simulink model "kalman_estimate_MM"  (R2018b)
settings: Solver=FixedStepAuto  StartTime=0.0  StopTime=500  FixedStep=0.02  RelTol=1e-3
values from neighbouring files (symbols this model uses):
  D = randn(num_output,num_control)    [Com_of_linear_model_calculate.m]    (also in Copy_of_linear_model_calculate.m; D.mat = [0 0 0.00507528406191 0.0236369284061 0.221173094143 0.00198; LINEAR.m = randn(8,1)*10; MM_HKF.m = reshape(out(A_l+B_l+C_l+1:A_l+B_l+C_l+D_l),size_D))
undefined symbols (not defined in the file or in its folder): act_piece, com_piece, piece, sigbuilder_block
libraries: sharedschedule x467, dspsigattribs x44, commchan3 x1
(part 3 of 5)

== system kalman_estimate_MM/HKF8 ==
  In3 : Inport
  In4 : Inport  Port=2
  x_obem : Inport  Port=3
  y_obem : Inport  Port=4
  A : sharedschedule/Interpolate Matrix(x)   matrix=piece.A  aMode=aMode
      settings: SourceProductName=Aerospace Blockset  SourceProductBaseCode=AE
  Add : Sum
  B : sharedschedule/Interpolate Matrix(x)   matrix=piece.B  aMode=aMode
      settings: SourceProductName=Aerospace Blockset  SourceProductBaseCode=AE
  C : sharedschedule/Interpolate Matrix(x)   matrix=piece.C  aMode=aMode
      settings: SourceProductName=Aerospace Blockset  SourceProductBaseCode=AE
  D : sharedschedule/Interpolate Matrix(x)   matrix=piece.D  aMode=aMode
      settings: SourceProductName=Aerospace Blockset  SourceProductBaseCode=AE
  K_s : sharedschedule/Interpolate Matrix(x)   matrix=piece.K_s  aMode=aMode
      settings: SourceProductName=Aerospace Blockset  SourceProductBaseCode=AE
  L : sharedschedule/Interpolate Matrix(x)   matrix=piece.L  aMode=aMode
      settings: SourceProductName=Aerospace Blockset  SourceProductBaseCode=AE
  M : sharedschedule/Interpolate Matrix(x)   matrix=piece.M  aMode=aMode
      settings: SourceProductName=Aerospace Blockset  SourceProductBaseCode=AE
  Prelookup : PreLookup  BreakpointsData=piece.Nl  BreakpointObject=Nl  ExtrapMethod=Linear  UseLastBreakpoint=on  DiagnosticForOutOfRangeInput=Warning
  S : sharedschedule/Interpolate Matrix(x)   matrix=piece.S_s  aMode=aMode
      settings: SourceProductName=Aerospace Blockset  SourceProductBaseCode=AE
  Selector : Selector  InputPortWidth=2  IndexOptions=Index vector (dialog)  Indices=[1]  OutputSizes=1
  kalman filter1 : Subsystem
  steadyOutput : sharedschedule/Interpolate Matrix(x)   matrix=piece.steadyOutput  aMode=aMode
      settings: SourceProductName=Aerospace Blockset  SourceProductBaseCode=AE
  steadyState : sharedschedule/Interpolate Matrix(x)   matrix=piece.steadyState  aMode=aMode
      settings: SourceProductName=Aerospace Blockset  SourceProductBaseCode=AE
  steadyinput : sharedschedule/Interpolate Matrix(x)   matrix=piece.steadyInput  aMode=aMode
      settings: SourceProductName=Aerospace Blockset  SourceProductBaseCode=AE
  Out1 : Outport
  Out2 : Outport  Port=2
  wires:
  Prelookup/1 -> S/1, K_s/1, M/1, L/1, steadyState/1, steadyinput/1, steadyOutput/1, D/1, C/1, B/1, A/1
  In4/1 -> kalman filter1/7(P)
  Prelookup/2 -> A/2, steadyState/2, S/2, K_s/2, M/2, L/2, steadyinput/2, steadyOutput/2, D/2, C/2, B/2
  Selector/1 -> Prelookup/1
  L/1 -> kalman filter1/5(L)
  C/1 -> kalman filter1/2(C)
  kalman filter1/1(X_es) -> Selector/1
  A/1 -> kalman filter1/1(A)
  M/1 -> kalman filter1/6(M)
  In3/1 -> kalman filter1/3(x0)
  x_obem/1 -> kalman filter1/4(Xtrim)
  y_obem/1 -> Add/2
  kalman filter1/2(Y_es) -> Add/1, Out1/1
  Add/1 -> Out2/1

== system kalman_estimate_MM/HKF9 ==
  In2 : Inport
  In3 : Inport  Port=2
  In4 : Inport  Port=3
  x_obem : Inport  Port=4
  y_obem : Inport  Port=5
  A : sharedschedule/Interpolate Matrix(x)   matrix=piece.A  aMode=aMode
      settings: SourceProductName=Aerospace Blockset  SourceProductBaseCode=AE
  B : sharedschedule/Interpolate Matrix(x)   matrix=piece.B  aMode=aMode
      settings: SourceProductName=Aerospace Blockset  SourceProductBaseCode=AE
  C : sharedschedule/Interpolate Matrix(x)   matrix=piece.C  aMode=aMode
      settings: SourceProductName=Aerospace Blockset  SourceProductBaseCode=AE
  D : sharedschedule/Interpolate Matrix(x)   matrix=piece.D  aMode=aMode
      settings: SourceProductName=Aerospace Blockset  SourceProductBaseCode=AE
  K_s : sharedschedule/Interpolate Matrix(x)   matrix=piece.K_s  aMode=aMode
      settings: SourceProductName=Aerospace Blockset  SourceProductBaseCode=AE
  L : sharedschedule/Interpolate Matrix(x)   matrix=piece.L  aMode=aMode
      settings: SourceProductName=Aerospace Blockset  SourceProductBaseCode=AE
  M : sharedschedule/Interpolate Matrix(x)   matrix=piece.M  aMode=aMode
      settings: SourceProductName=Aerospace Blockset  SourceProductBaseCode=AE
  MATLAB Function : MATLAB Function  TreatAsAtomicUnit=on
  Minus5 : Sum  Inputs=+-
  Prelookup : PreLookup  BreakpointsData=piece.Nl  BreakpointObject=Nl  ExtrapMethod=Linear  UseLastBreakpoint=on  DiagnosticForOutOfRangeInput=Warning
  S : sharedschedule/Interpolate Matrix(x)   matrix=piece.S_s  aMode=aMode
      settings: SourceProductName=Aerospace Blockset  SourceProductBaseCode=AE
  Selector : Selector  InputPortWidth=2  IndexOptions=Index vector (dialog)  Indices=[1]  OutputSizes=1
  kalman filter1 : Subsystem
  steadyOutput : sharedschedule/Interpolate Matrix(x)   matrix=piece.steadyOutput  aMode=aMode
      settings: SourceProductName=Aerospace Blockset  SourceProductBaseCode=AE
  steadyState : sharedschedule/Interpolate Matrix(x)   matrix=piece.steadyState  aMode=aMode
      settings: SourceProductName=Aerospace Blockset  SourceProductBaseCode=AE
  steadyinput : sharedschedule/Interpolate Matrix(x)   matrix=piece.steadyInput  aMode=aMode
      settings: SourceProductName=Aerospace Blockset  SourceProductBaseCode=AE
  Out1 : Outport
  Out2 : Outport  Port=2
  Out3 : Outport  Port=3
  wires:
  S/1 -> MATLAB Function/2(S)
  kalman filter1/3(Y_error) -> Out2/1, MATLAB Function/1(err)
  MATLAB Function/1(y) -> Out3/1
  Prelookup/1 -> S/1, K_s/1, M/1, L/1, steadyState/1, steadyinput/1, steadyOutput/1, D/1, C/1, B/1, A/1
  In4/1 -> kalman filter1/9(P)
  Prelookup/2 -> A/2, steadyState/2, S/2, K_s/2, M/2, L/2, steadyinput/2, steadyOutput/2, D/2, C/2, B/2
  Selector/1 -> Prelookup/1
  L/1 -> kalman filter1/7(L)
  C/1 -> kalman filter1/2(C)
  Minus5/1 -> kalman filter1/5(Y)
  kalman filter1/2(Y_es) -> Out1/1
  kalman filter1/1(X_es) -> Selector/1
  K_s/1 -> kalman filter1/3(K)
  A/1 -> kalman filter1/1(A)
  M/1 -> kalman filter1/8(M)
  In3/1 -> kalman filter1/4(x0)
  In2/1 -> Minus5/1
  y_obem/1 -> Minus5/2
  x_obem/1 -> kalman filter1/6(Xtrim)

== system kalman_estimate_MM/PIECE kalman ==
  In1 : Inport
  In2 : Inport  Port=2
  In3 : Inport  Port=3
  In4 : Inport  Port=4
  A : sharedschedule/Interpolate Matrix(x)   matrix=piece.A  aMode=aMode
      settings: SourceProductName=Aerospace Blockset  SourceProductBaseCode=AE
  B : sharedschedule/Interpolate Matrix(x)   matrix=piece.B  aMode=aMode
      settings: SourceProductName=Aerospace Blockset  SourceProductBaseCode=AE
  C : sharedschedule/Interpolate Matrix(x)   matrix=piece.C  aMode=aMode
      settings: SourceProductName=Aerospace Blockset  SourceProductBaseCode=AE
  D : sharedschedule/Interpolate Matrix(x)   matrix=piece.D  aMode=aMode
      settings: SourceProductName=Aerospace Blockset  SourceProductBaseCode=AE
  K_s : sharedschedule/Interpolate Matrix(x)   matrix=piece.K_s  aMode=aMode
      settings: SourceProductName=Aerospace Blockset  SourceProductBaseCode=AE
  L : sharedschedule/Interpolate Matrix(x)   matrix=piece.L  aMode=aMode
      settings: SourceProductName=Aerospace Blockset  SourceProductBaseCode=AE
  M : sharedschedule/Interpolate Matrix(x)   matrix=piece.M  aMode=aMode
      settings: SourceProductName=Aerospace Blockset  SourceProductBaseCode=AE
  Minus1 : Sum  Inputs=+-
  Minus5 : Sum  Inputs=+-
  Prelookup : PreLookup  BreakpointsData=piece.Nl  BreakpointObject=Nl  ExtrapMethod=Linear  UseLastBreakpoint=on  DiagnosticForOutOfRangeInput=Warning
  S : sharedschedule/Interpolate Matrix(x)   matrix=piece.S_s  aMode=aMode
      settings: SourceProductName=Aerospace Blockset  SourceProductBaseCode=AE
  Selector : Selector  InputPortWidth=2  IndexOptions=Index vector (dialog)  Indices=[1]  OutputSizes=1
  kalman filter1 : Subsystem
  steadyOutput : sharedschedule/Interpolate Matrix(x)   matrix=piece.steadyOutput  aMode=aMode
      settings: SourceProductName=Aerospace Blockset  SourceProductBaseCode=AE
  steadyState : sharedschedule/Interpolate Matrix(x)   matrix=piece.steadyState  aMode=aMode
      settings: SourceProductName=Aerospace Blockset  SourceProductBaseCode=AE
  steadyinput : sharedschedule/Interpolate Matrix(x)   matrix=piece.steadyInput  aMode=aMode
      settings: SourceProductName=Aerospace Blockset  SourceProductBaseCode=AE
  Out1 : Outport
  Out2 : Outport  Port=2
  wires:
  kalman filter1/3(Y_error) -> Out2/1
  In1/1 -> Minus1/1
  In2/1 -> Minus5/1
  In3/1 -> kalman filter1/6(x0)
  M/1 -> kalman filter1/11(M)
  A/1 -> kalman filter1/1(A)
  steadyOutput/1 -> Minus5/2
  K_s/1 -> kalman filter1/5(K)
  steadyinput/1 -> Minus1/2
  kalman filter1/1(X_es) -> Selector/1
  Minus1/1 -> kalman filter1/8(U)
  kalman filter1/2(Y_es) -> Out1/1
  Minus5/1 -> kalman filter1/7(Y)
  C/1 -> kalman filter1/3(C)
  L/1 -> kalman filter1/10(L)
  steadyState/1 -> kalman filter1/9(Xtrim)
  Selector/1 -> Prelookup/1
  Prelookup/2 -> B/2, C/2, D/2, steadyOutput/2, steadyinput/2, L/2, M/2, K_s/2, S/2, steadyState/2, A/2
  B/1 -> kalman filter1/2(B)
  In4/1 -> kalman filter1/12(P)
  Prelookup/1 -> A/1, B/1, C/1, D/1, steadyOutput/1, steadyinput/1, steadyState/1, L/1, M/1, K_s/1, S/1
  D/1 -> kalman filter1/4(D)

== system kalman_estimate_MM/PIECE kalman1 ==
  u : Inport
  y : Inport  Port=2
  x0 : Inport  Port=3
  hp : Inport  Port=4
  A : sharedschedule/Interpolate Matrix(x)   matrix=piece.A  aMode=aMode
      settings: SourceProductName=Aerospace Blockset  SourceProductBaseCode=AE
  B : sharedschedule/Interpolate Matrix(x)   matrix=piece.B  aMode=aMode
      settings: SourceProductName=Aerospace Blockset  SourceProductBaseCode=AE
  C : sharedschedule/Interpolate Matrix(x)   matrix=piece.C  aMode=aMode
      settings: SourceProductName=Aerospace Blockset  SourceProductBaseCode=AE
  D : sharedschedule/Interpolate Matrix(x)   matrix=piece.D  aMode=aMode
      settings: SourceProductName=Aerospace Blockset  SourceProductBaseCode=AE
  K_s : sharedschedule/Interpolate Matrix(x)   matrix=piece.K_s  aMode=aMode
      settings: SourceProductName=Aerospace Blockset  SourceProductBaseCode=AE
  L : sharedschedule/Interpolate Matrix(x)   matrix=piece.L  aMode=aMode
      settings: SourceProductName=Aerospace Blockset  SourceProductBaseCode=AE
  M : sharedschedule/Interpolate Matrix(x)   matrix=piece.M  aMode=aMode
      settings: SourceProductName=Aerospace Blockset  SourceProductBaseCode=AE
  MATLAB Function : MATLAB Function  TreatAsAtomicUnit=on
  Minus1 : Sum  Inputs=+-
  Minus5 : Sum  Inputs=+-
  Prelookup : PreLookup  BreakpointsData=piece.Nl  BreakpointObject=Nl  ExtrapMethod=Linear  UseLastBreakpoint=on  DiagnosticForOutOfRangeInput=Warning
  S : sharedschedule/Interpolate Matrix(x)   matrix=piece.S_s  aMode=aMode
      settings: SourceProductName=Aerospace Blockset  SourceProductBaseCode=AE
  Selector : Selector  InputPortWidth=2  IndexOptions=Index vector (dialog)  Indices=[1]  OutputSizes=1
  kalman filter1 : Subsystem
  steadyOutput : sharedschedule/Interpolate Matrix(x)   matrix=piece.steadyOutput  aMode=aMode
      settings: SourceProductName=Aerospace Blockset  SourceProductBaseCode=AE
  steadyState : sharedschedule/Interpolate Matrix(x)   matrix=piece.steadyState  aMode=aMode
      settings: SourceProductName=Aerospace Blockset  SourceProductBaseCode=AE
  steadyinput : sharedschedule/Interpolate Matrix(x)   matrix=piece.steadyInput  aMode=aMode
      settings: SourceProductName=Aerospace Blockset  SourceProductBaseCode=AE
  Out1 : Outport
  Out2 : Outport  Port=2
  Out3 : Outport  Port=3
  wires:
  u/1 -> Minus1/1
  y/1 -> Minus5/1
  x0/1 -> kalman filter1/6(x0)
  M/1 -> kalman filter1/11(M)
  A/1 -> kalman filter1/1(A)
  steadyOutput/1 -> Minus5/2
  K_s/1 -> kalman filter1/5(K)
  steadyinput/1 -> Minus1/2
  kalman filter1/1(X_es) -> Selector/1
  Minus1/1 -> kalman filter1/8(U)
  kalman filter1/2(Y_es) -> Out1/1
  Minus5/1 -> kalman filter1/7(Y)
  C/1 -> kalman filter1/3(C)
  L/1 -> kalman filter1/10(L)
  steadyState/1 -> kalman filter1/9(Xtrim)
  Selector/1 -> Prelookup/1
  Prelookup/2 -> B/2, C/2, D/2, steadyOutput/2, steadyinput/2, L/2, M/2, K_s/2, S/2, steadyState/2, A/2
  B/1 -> kalman filter1/2(B)
  hp/1 -> kalman filter1/12(P)
  Prelookup/1 -> A/1, B/1, C/1, D/1, steadyOutput/1, steadyinput/1, steadyState/1, L/1, M/1, K_s/1, S/1
  D/1 -> kalman filter1/4(D)
  S/1 -> MATLAB Function/2(S)
  kalman filter1/3(Y_error) -> MATLAB Function/1(err), Out2/1
  MATLAB Function/1(y) -> Out3/1

== system kalman_estimate_MM/PWL ==
  In1 : Inport
  In3 : Inport  Port=2
  In4 : Inport  Port=3
  A : sharedschedule/Interpolate Matrix(x)   matrix=piece.A  aMode=aMode
      settings: SourceProductName=Aerospace Blockset  SourceProductBaseCode=AE
  Add : Sum
  B : sharedschedule/Interpolate Matrix(x)   matrix=piece.B  aMode=aMode
      settings: SourceProductName=Aerospace Blockset  SourceProductBaseCode=AE
  C : sharedschedule/Interpolate Matrix(x)   matrix=piece.C  aMode=aMode
      settings: SourceProductName=Aerospace Blockset  SourceProductBaseCode=AE
  D : sharedschedule/Interpolate Matrix(x)   matrix=piece.D  aMode=aMode
      settings: SourceProductName=Aerospace Blockset  SourceProductBaseCode=AE
  K_s : sharedschedule/Interpolate Matrix(x)   matrix=piece.K_s  aMode=aMode
      settings: SourceProductName=Aerospace Blockset  SourceProductBaseCode=AE
  L : sharedschedule/Interpolate Matrix(x)   matrix=piece.L  aMode=aMode
      settings: SourceProductName=Aerospace Blockset  SourceProductBaseCode=AE
  M : sharedschedule/Interpolate Matrix(x)   matrix=piece.M  aMode=aMode
      settings: SourceProductName=Aerospace Blockset  SourceProductBaseCode=AE
  Minus1 : Sum  Inputs=+-
  Prelookup : PreLookup  BreakpointsData=piece.Nl  BreakpointObject=Nl  ExtrapMethod=Linear  UseLastBreakpoint=on  DiagnosticForOutOfRangeInput=Warning
  S : sharedschedule/Interpolate Matrix(x)   matrix=piece.S_s  aMode=aMode
      settings: SourceProductName=Aerospace Blockset  SourceProductBaseCode=AE
  Selector : Selector  InputPortWidth=2  IndexOptions=Index vector (dialog)  Indices=[1]  OutputSizes=1
  kalman filter1 : Subsystem
  steadyOutput : sharedschedule/Interpolate Matrix(x)   matrix=piece.steadyOutput  aMode=aMode
      settings: SourceProductName=Aerospace Blockset  SourceProductBaseCode=AE
  steadyState : sharedschedule/Interpolate Matrix(x)   matrix=piece.steadyState  aMode=aMode
      settings: SourceProductName=Aerospace Blockset  SourceProductBaseCode=AE
  steadyinput : sharedschedule/Interpolate Matrix(x)   matrix=piece.steadyInput  aMode=aMode
      settings: SourceProductName=Aerospace Blockset  SourceProductBaseCode=AE
  Out1 : Outport
  Out2 : Outport  Port=2
  wires:
  D/1 -> kalman filter1/4(D)
  Prelookup/1 -> S/1, K_s/1, M/1, L/1, steadyState/1, steadyinput/1, steadyOutput/1, D/1, C/1, B/1, A/1
  In4/1 -> kalman filter1/11(P)
  B/1 -> kalman filter1/2(B)
  Prelookup/2 -> A/2, steadyState/2, S/2, K_s/2, M/2, L/2, steadyinput/2, steadyOutput/2, D/2, C/2, B/2
  Selector/1 -> Prelookup/1
  steadyState/1 -> kalman filter1/8(Xtrim)
  L/1 -> kalman filter1/9(L)
  C/1 -> kalman filter1/3(C)
  kalman filter1/2(Y_es) -> Add/1, Out1/1
  Minus1/1 -> kalman filter1/7(U)
  kalman filter1/1(X_es) -> Selector/1
  steadyinput/1 -> Minus1/2
  K_s/1 -> kalman filter1/5(K)
  A/1 -> kalman filter1/1(A)
  M/1 -> kalman filter1/10(M)
  In3/1 -> kalman filter1/6(x0)
  In1/1 -> Minus1/1
  steadyOutput/1 -> Add/2
  Add/1 -> Out2/1

== system kalman_estimate_MM/Signal Builder ==
  Demux : Demux  Tag=STV Demux  Outputs=6
  FromWs : FromWorkspace  Tag=STV FromWs  VariableName=tuvar  SampleTime=0
      SigBuilderData=|
      | common.afterFinalStr = 'Extrapolate'
      | common.sampleTime = 0
      | dataSet.timeRange = [0 500]
      | dataSet.name = 'Group 1'
      | sbobj.Groups.Name = 'Group 1'
      | sbobj.Groups.Signals(1).Name = 'Signal 2'
      | sbobj.Groups.Signals(1).XData = [0 120 120 500]
      | sbobj.Groups.Signals(1).YData = [0 0 -0.02 -0.02]
      | sbobj.Groups.Signals(2).Name = 'Signal 3'
      | sbobj.Groups.Signals(2).XData = [0 135 170 500]
      | sbobj.Groups.Signals(2).YData = [0 0 0 0]
      | sbobj.Groups.Signals(3).Name = 'Signal 4'
      | sbobj.Groups.Signals(3).XData = [0 135 170 500]
      | sbobj.Groups.Signals(3).YData = [0 0 0 0]
      | sbobj.Groups.Signals(4).Name = 'Signal 1'
      | sbobj.Groups.Signals(4).XData = [0 135 170 500]
      | sbobj.Groups.Signals(4).YData = [0 0 0 0]
      | sbobj.Groups.Signals(5).Name = 'Signal 5'
      | sbobj.Groups.Signals(5).XData = [0 135 170 500]
      | sbobj.Groups.Signals(5).YData = [0 0 0 0]
      | sbobj.Groups.Signals(6).Name = 'Signal 6'
      | sbobj.Groups.Signals(6).XData = [0 135 170 500]
      | sbobj.Groups.Signals(6).YData = [0 0 0 0]
      | sbobj.Groups.TimeRange = [0 500]
  Signal 2 : Outport  Tag=STV Outport
  Signal 3 : Outport  Tag=STV Outport  Port=2
  Signal 4 : Outport  Tag=STV Outport  Port=3
  Signal 1 : Outport  Tag=STV Outport  Port=4
  Signal 5 : Outport  Tag=STV Outport  Port=5
  Signal 6 : Outport  Tag=STV Outport  Port=6
  wires:
  FromWs/1 -> Demux/1
  Demux/1 -> Signal 2/1
  Demux/2 -> Signal 3/1
  Demux/3 -> Signal 4/1
  Demux/4 -> Signal 1/1
  Demux/5 -> Signal 5/1
  Demux/6 -> Signal 6/1

== system kalman_estimate_MM/Signal Builder1 ==
  Demux : Demux  Tag=STV Demux  Outputs=6
  FromWs : FromWorkspace  Tag=STV FromWs  VariableName=tuvar  SampleTime=0
      SigBuilderData=|
      | common.afterFinalStr = 'Extrapolate'
      | common.sampleTime = 0
      | dataSet.timeRange = [0 500]
      | dataSet.name = 'Group 1'
      | sbobj.Groups.Name = 'Group 1'
      | sbobj.Groups.Signals(1).Name = 'Signal 2'
      | sbobj.Groups.Signals(1).XData = [0 135 170 500]
      | sbobj.Groups.Signals(1).YData = [0 0 0 0]
      | sbobj.Groups.Signals(2).Name = 'Signal 3'
      | sbobj.Groups.Signals(2).XData = [0 50 50 500]
      | sbobj.Groups.Signals(2).YData = [0 0 -0.02 -0.02]
      | sbobj.Groups.Signals(3).Name = 'Signal 4'
      | sbobj.Groups.Signals(3).XData = [0 135 170 500]
      | sbobj.Groups.Signals(3).YData = [0 0 0 0]
      | sbobj.Groups.Signals(4).Name = 'Signal 1'
      | sbobj.Groups.Signals(4).XData = [0 120 120 500]
      | sbobj.Groups.Signals(4).YData = [0 0 -0.02 -0.02]
      | sbobj.Groups.Signals(5).Name = 'Signal 5'
      | sbobj.Groups.Signals(5).XData = [0 200 200 500]
      | sbobj.Groups.Signals(5).YData = [0 0 -0.02 -0.02]
      | sbobj.Groups.Signals(6).Name = 'Signal 6'
      | sbobj.Groups.Signals(6).XData = [0 135 170 500]
      | sbobj.Groups.Signals(6).YData = [0 0 0 0]
      | sbobj.Groups.TimeRange = [0 500]
  Signal 2 : Outport  Tag=STV Outport
  Signal 3 : Outport  Tag=STV Outport  Port=2
  Signal 4 : Outport  Tag=STV Outport  Port=3
  Signal 1 : Outport  Tag=STV Outport  Port=4
  Signal 5 : Outport  Tag=STV Outport  Port=5
  Signal 6 : Outport  Tag=STV Outport  Port=6
  wires:
  Demux/6 -> Signal 6/1
  Demux/5 -> Signal 5/1
  Demux/4 -> Signal 1/1
  Demux/3 -> Signal 4/1
  Demux/2 -> Signal 3/1
  Demux/1 -> Signal 2/1
  FromWs/1 -> Demux/1

== system kalman_estimate_MM/act_PIECE kalman ==
  u : Inport
  y : Inport  Port=2
  x0 : Inport  Port=3
  A : sharedschedule/Interpolate Matrix(x)   matrix=act_piece.A  aMode=aMode
      settings: SourceProductName=Aerospace Blockset  SourceProductBaseCode=AE
  B : sharedschedule/Interpolate Matrix(x)   matrix=act_piece.B  aMode=aMode
      settings: SourceProductName=Aerospace Blockset  SourceProductBaseCode=AE
  C : sharedschedule/Interpolate Matrix(x)   matrix=act_piece.C  aMode=aMode
      settings: SourceProductName=Aerospace Blockset  SourceProductBaseCode=AE
  D : sharedschedule/Interpolate Matrix(x)   matrix=act_piece.D  aMode=aMode
      settings: SourceProductName=Aerospace Blockset  SourceProductBaseCode=AE
  K_s : sharedschedule/Interpolate Matrix(x)   matrix=act_piece.K  aMode=aMode
      settings: SourceProductName=Aerospace Blockset  SourceProductBaseCode=AE
  MATLAB Function : MATLAB Function  TreatAsAtomicUnit=on
  Minus1 : Sum  Inputs=+-
  Minus5 : Sum  Inputs=+-
  Prelookup : PreLookup  BreakpointsData=act_piece.Nl  BreakpointObject=Nl  ExtrapMethod=Linear  UseLastBreakpoint=on  DiagnosticForOutOfRangeInput=Warning
  S : sharedschedule/Interpolate Matrix(x)   matrix=act_piece.S  aMode=aMode
      settings: SourceProductName=Aerospace Blockset  SourceProductBaseCode=AE
  Selector : Selector  InputPortWidth=2  IndexOptions=Index vector (dialog)  Indices=[1]  OutputSizes=1
  kalman filter1 : Subsystem
  steadyOutput : sharedschedule/Interpolate Matrix(x)   matrix=act_piece.steadyOutput  aMode=aMode
      settings: SourceProductName=Aerospace Blockset  SourceProductBaseCode=AE
  steadyState : sharedschedule/Interpolate Matrix(x)   matrix=act_piece.steadyState  aMode=aMode
      settings: SourceProductName=Aerospace Blockset  SourceProductBaseCode=AE
  steadyinput : sharedschedule/Interpolate Matrix(x)   matrix=piece.steadyInput  aMode=aMode
      settings: SourceProductName=Aerospace Blockset  SourceProductBaseCode=AE
  Out1 : Outport
  Out2 : Outport  Port=2
  Out3 : Outport  Port=3
  wires:
  kalman filter1/3(Y_error) -> MATLAB Function/1(err), Out2/1
  u/1 -> Minus1/1
  y/1 -> Minus5/1
  x0/1 -> kalman filter1/6(x0)
  A/1 -> kalman filter1/1(A)
  steadyOutput/1 -> Minus5/2
  K_s/1 -> kalman filter1/5(K)
  steadyinput/1 -> Minus1/2
  kalman filter1/1(X_es) -> Selector/1
  Minus1/1 -> kalman filter1/8(U)
  kalman filter1/2(Y_es) -> Out1/1
  Minus5/1 -> kalman filter1/7(Y)
  C/1 -> kalman filter1/3(C)
  steadyState/1 -> kalman filter1/9(Xtrim)
  Selector/1 -> Prelookup/1
  Prelookup/2 -> B/2, C/2, D/2, steadyOutput/2, steadyinput/2, K_s/2, S/2, steadyState/2, A/2
  B/1 -> kalman filter1/2(B)
  Prelookup/1 -> A/1, B/1, C/1, D/1, steadyOutput/1, steadyinput/1, steadyState/1, S/1, K_s/1
  D/1 -> kalman filter1/4(D)
  S/1 -> MATLAB Function/2(S)
  MATLAB Function/1(y) -> Out3/1

== system kalman_estimate_MM/act_PWL ==
  u : Inport
  x0 : Inport  Port=2
  A : sharedschedule/Interpolate Matrix(x)   matrix=act_piece.A  aMode=aMode
      settings: SourceProductName=Aerospace Blockset  SourceProductBaseCode=AE
  Add : Sum
  B : sharedschedule/Interpolate Matrix(x)   matrix=act_piece.B  aMode=aMode
      settings: SourceProductName=Aerospace Blockset  SourceProductBaseCode=AE
  C : sharedschedule/Interpolate Matrix(x)   matrix=act_piece.C  aMode=aMode
      settings: SourceProductName=Aerospace Blockset  SourceProductBaseCode=AE
  D : sharedschedule/Interpolate Matrix(x)   matrix=act_piece.D  aMode=aMode
      settings: SourceProductName=Aerospace Blockset  SourceProductBaseCode=AE
  K : sharedschedule/Interpolate Matrix(x)   matrix=act_piece.K  aMode=aMode
      settings: SourceProductName=Aerospace Blockset  SourceProductBaseCode=AE
  Minus1 : Sum  Inputs=+-
  Prelookup : PreLookup  BreakpointsData=act_piece.Nl  BreakpointObject=Nl  ExtrapMethod=Linear  UseLastBreakpoint=on  DiagnosticForOutOfRangeInput=Warning
  S : sharedschedule/Interpolate Matrix(x)   matrix=act_piece.S  aMode=aMode
      settings: SourceProductName=Aerospace Blockset  SourceProductBaseCode=AE
  Selector : Selector  InputPortWidth=2  IndexOptions=Index vector (dialog)  Indices=[1]  OutputSizes=1
  kalman filter1 : Subsystem
  steadyOutput : sharedschedule/Interpolate Matrix(x)   matrix=act_piece.steadyOutput  aMode=aMode
      settings: SourceProductName=Aerospace Blockset  SourceProductBaseCode=AE
  steadyState : sharedschedule/Interpolate Matrix(x)   matrix=act_piece.steadyState  aMode=aMode
      settings: SourceProductName=Aerospace Blockset  SourceProductBaseCode=AE
  steadyinput : sharedschedule/Interpolate Matrix(x)   matrix=act_piece.steadyInput  aMode=aMode
      settings: SourceProductName=Aerospace Blockset  SourceProductBaseCode=AE
  Out1 : Outport
  Out2 : Outport  Port=2
  wires:
  Add/1 -> Out2/1
  steadyOutput/1 -> Add/2
  u/1 -> Minus1/1
  x0/1 -> kalman filter1/5(x0)
  A/1 -> kalman filter1/1(A)
  steadyinput/1 -> Minus1/2
  kalman filter1/1(X_es) -> Selector/1
  Minus1/1 -> kalman filter1/6(U)
  kalman filter1/2(Y_es) -> Out1/1, Add/1
  C/1 -> kalman filter1/3(C)
  steadyState/1 -> kalman filter1/7(Xtrim)
  Selector/1 -> Prelookup/1
  Prelookup/2 -> B/2, C/2, D/2, steadyOutput/2, steadyinput/2, K/2, S/2, steadyState/2, A/2
  B/1 -> kalman filter1/2(B)
  Prelookup/1 -> A/1, B/1, C/1, D/1, steadyOutput/1, steadyinput/1, steadyState/1, K/1, S/1
  D/1 -> kalman filter1/4(D)

== system kalman_estimate_MM/act_PWL_model ==
  u : Inport
  x0 : Inport  Port=2
  A : sharedschedule/Interpolate Matrix(x)   matrix=act_piece.A  aMode=aMode
      settings: SourceProductName=Aerospace Blockset  SourceProductBaseCode=AE
  Add : Sum
  B : sharedschedule/Interpolate Matrix(x)   matrix=act_piece.B  aMode=aMode
      settings: SourceProductName=Aerospace Blockset  SourceProductBaseCode=AE
  C : sharedschedule/Interpolate Matrix(x)   matrix=act_piece.C  aMode=aMode
      settings: SourceProductName=Aerospace Blockset  SourceProductBaseCode=AE
  D : sharedschedule/Interpolate Matrix(x)   matrix=act_piece.D  aMode=aMode
      settings: SourceProductName=Aerospace Blockset  SourceProductBaseCode=AE
  K : sharedschedule/Interpolate Matrix(x)   matrix=act_piece.K  aMode=aMode
      settings: SourceProductName=Aerospace Blockset  SourceProductBaseCode=AE
  Minus1 : Sum  Inputs=+-
  Prelookup : PreLookup  BreakpointsData=piece.Nl  BreakpointObject=Nl  ExtrapMethod=Linear  UseLastBreakpoint=on  DiagnosticForOutOfRangeInput=Warning
  S : sharedschedule/Interpolate Matrix(x)   matrix=act_piece.S  aMode=aMode
      settings: SourceProductName=Aerospace Blockset  SourceProductBaseCode=AE
  Selector : Selector  InputPortWidth=2  IndexOptions=Index vector (dialog)  Indices=[1]  OutputSizes=1
  kalman filter1 : Subsystem
  steadyOutput : sharedschedule/Interpolate Matrix(x)   matrix=act_piece.steadyOutput  aMode=aMode
      settings: SourceProductName=Aerospace Blockset  SourceProductBaseCode=AE
  steadyState : sharedschedule/Interpolate Matrix(x)   matrix=act_piece.steadyState  aMode=aMode
      settings: SourceProductName=Aerospace Blockset  SourceProductBaseCode=AE
  steadyinput : sharedschedule/Interpolate Matrix(x)   matrix=piece.steadyInput  aMode=aMode
      settings: SourceProductName=Aerospace Blockset  SourceProductBaseCode=AE
  Out1 : Outport
  Out2 : Outport  Port=2
  wires:
  D/1 -> kalman filter1/4(D)
  Prelookup/1 -> S/1, K/1, steadyState/1, steadyinput/1, steadyOutput/1, D/1, C/1, B/1, A/1
  B/1 -> kalman filter1/2(B)
  Prelookup/2 -> A/2, steadyState/2, S/2, K/2, steadyinput/2, steadyOutput/2, D/2, C/2, B/2
  Selector/1 -> Prelookup/1
  steadyState/1 -> kalman filter1/7(Xtrim)
  C/1 -> kalman filter1/3(C)
  kalman filter1/2(Y_es) -> Add/1, Out1/1
  Minus1/1 -> kalman filter1/6(U)
  kalman filter1/1(X_es) -> Selector/1
  steadyinput/1 -> Minus1/2
  A/1 -> kalman filter1/1(A)
  x0/1 -> kalman filter1/5(x0)
  u/1 -> Minus1/1
  steadyOutput/1 -> Add/2
  Add/1 -> Out2/1

== system kalman_estimate_MM/com_PIECE kalman ==
  u : Inport
  y : Inport  Port=2
  x0 : Inport  Port=3
  A : sharedschedule/Interpolate Matrix(x)   matrix=com_piece.A  aMode=aMode
      settings: SourceProductName=Aerospace Blockset  SourceProductBaseCode=AE
  B : sharedschedule/Interpolate Matrix(x)   matrix=com_piece.B  aMode=aMode
      settings: SourceProductName=Aerospace Blockset  SourceProductBaseCode=AE
  C : sharedschedule/Interpolate Matrix(x)   matrix=com_piece.C  aMode=aMode
      settings: SourceProductName=Aerospace Blockset  SourceProductBaseCode=AE
  D : sharedschedule/Interpolate Matrix(x)   matrix=com_piece.D  aMode=aMode
      settings: SourceProductName=Aerospace Blockset  SourceProductBaseCode=AE
  K_s : sharedschedule/Interpolate Matrix(x)   matrix=com_piece.K  aMode=aMode
      settings: SourceProductName=Aerospace Blockset  SourceProductBaseCode=AE
  MATLAB Function : MATLAB Function  TreatAsAtomicUnit=on
  Minus1 : Sum  Inputs=+-
  Minus5 : Sum  Inputs=+-
  Prelookup : PreLookup  BreakpointsData=com_piece.Nl  BreakpointObject=Nl  ExtrapMethod=Linear  UseLastBreakpoint=on  DiagnosticForOutOfRangeInput=Warning
  S : sharedschedule/Interpolate Matrix(x)   matrix=com_piece.S  aMode=aMode
      settings: SourceProductName=Aerospace Blockset  SourceProductBaseCode=AE
  Selector : Selector  InputPortWidth=2  IndexOptions=Index vector (dialog)  Indices=[1]  OutputSizes=1
  kalman filter1 : Subsystem
  steadyOutput : sharedschedule/Interpolate Matrix(x)   matrix=com_piece.steadyOutput  aMode=aMode
      settings: SourceProductName=Aerospace Blockset  SourceProductBaseCode=AE
  steadyState : sharedschedule/Interpolate Matrix(x)   matrix=com_piece.steadyState  aMode=aMode
      settings: SourceProductName=Aerospace Blockset  SourceProductBaseCode=AE
  steadyinput : sharedschedule/Interpolate Matrix(x)   matrix=com_piece.steadyInput  aMode=aMode
      settings: SourceProductName=Aerospace Blockset  SourceProductBaseCode=AE
  Out1 : Outport
  Out2 : Outport  Port=2
  Out3 : Outport  Port=3
  wires:
  kalman filter1/3(Y_error) -> MATLAB Function/1(err), Out2/1
  u/1 -> Minus1/1
  y/1 -> Minus5/1
  x0/1 -> kalman filter1/6(x0)
  A/1 -> kalman filter1/1(A)
  steadyOutput/1 -> Minus5/2
  K_s/1 -> kalman filter1/5(K)
  steadyinput/1 -> Minus1/2
  kalman filter1/1(X_es) -> Selector/1
  Minus1/1 -> kalman filter1/8(U)
  kalman filter1/2(Y_es) -> Out1/1
  Minus5/1 -> kalman filter1/7(Y)
  C/1 -> kalman filter1/3(C)
  steadyState/1 -> kalman filter1/9(Xtrim)
  Selector/1 -> Prelookup/1
  Prelookup/2 -> B/2, C/2, D/2, steadyOutput/2, steadyinput/2, K_s/2, S/2, steadyState/2, A/2
  B/1 -> kalman filter1/2(B)
  Prelookup/1 -> A/1, B/1, C/1, D/1, steadyOutput/1, steadyinput/1, steadyState/1, K_s/1, S/1
  D/1 -> kalman filter1/4(D)
  S/1 -> MATLAB Function/2(S)
  MATLAB Function/1(y) -> Out3/1

== system kalman_estimate_MM/component_PWL ==
  u : Inport
  x0 : Inport  Port=2
  A : sharedschedule/Interpolate Matrix(x)   matrix=com_piece.A  aMode=aMode
      settings: SourceProductName=Aerospace Blockset  SourceProductBaseCode=AE
  Add : Sum
  B : sharedschedule/Interpolate Matrix(x)   matrix=com_piece.B  aMode=aMode
      settings: SourceProductName=Aerospace Blockset  SourceProductBaseCode=AE
  C : sharedschedule/Interpolate Matrix(x)   matrix=com_piece.C  aMode=aMode
      settings: SourceProductName=Aerospace Blockset  SourceProductBaseCode=AE
  D : sharedschedule/Interpolate Matrix(x)   matrix=com_piece.D  aMode=aMode
      settings: SourceProductName=Aerospace Blockset  SourceProductBaseCode=AE
  K : sharedschedule/Interpolate Matrix(x)   matrix=com_piece.K  aMode=aMode
      settings: SourceProductName=Aerospace Blockset  SourceProductBaseCode=AE
  Minus1 : Sum  Inputs=+-
  Prelookup : PreLookup  BreakpointsData=com_piece.Nl  BreakpointObject=Nl  ExtrapMethod=Linear  UseLastBreakpoint=on  DiagnosticForOutOfRangeInput=Warning
  S : sharedschedule/Interpolate Matrix(x)   matrix=com_piece.S  aMode=aMode
      settings: SourceProductName=Aerospace Blockset  SourceProductBaseCode=AE
  Selector : Selector  InputPortWidth=2  IndexOptions=Index vector (dialog)  Indices=[1]  OutputSizes=1
  kalman filter1 : Subsystem
  steadyOutput : sharedschedule/Interpolate Matrix(x)   matrix=com_piece.steadyOutput  aMode=aMode
      settings: SourceProductName=Aerospace Blockset  SourceProductBaseCode=AE
  steadyState : sharedschedule/Interpolate Matrix(x)   matrix=com_piece.steadyState  aMode=aMode
      settings: SourceProductName=Aerospace Blockset  SourceProductBaseCode=AE
  steadyinput : sharedschedule/Interpolate Matrix(x)   matrix=com_piece.steadyInput  aMode=aMode
      settings: SourceProductName=Aerospace Blockset  SourceProductBaseCode=AE
  Out1 : Outport
  Out2 : Outport  Port=2
  wires:
  Add/1 -> Out2/1
  steadyOutput/1 -> Add/2
  u/1 -> Minus1/1
  x0/1 -> kalman filter1/5(x0)
  A/1 -> kalman filter1/1(A)
  steadyinput/1 -> Minus1/2
  kalman filter1/1(X_es) -> Selector/1
  Minus1/1 -> kalman filter1/6(U)
  kalman filter1/2(Y_es) -> Out1/1, Add/1
  C/1 -> kalman filter1/3(C)
  steadyState/1 -> kalman filter1/7(Xtrim)
  Selector/1 -> Prelookup/1
  Prelookup/2 -> B/2, C/2, D/2, steadyOutput/2, steadyinput/2, K/2, S/2, steadyState/2, A/2
  B/1 -> kalman filter1/2(B)
  Prelookup/1 -> A/1, B/1, C/1, D/1, steadyOutput/1, steadyinput/1, steadyState/1, K/1, S/1
  D/1 -> kalman filter1/4(D)

== system kalman_estimate_MM/component_PWL1 ==
  u : Inport
  x0 : Inport  Port=2
  A : sharedschedule/Interpolate Matrix(x)   matrix=com_piece.A  aMode=aMode
      settings: SourceProductName=Aerospace Blockset  SourceProductBaseCode=AE
  Add : Sum
  B : sharedschedule/Interpolate Matrix(x)   matrix=com_piece.B  aMode=aMode
      settings: SourceProductName=Aerospace Blockset  SourceProductBaseCode=AE
  C : sharedschedule/Interpolate Matrix(x)   matrix=com_piece.C  aMode=aMode
      settings: SourceProductName=Aerospace Blockset  SourceProductBaseCode=AE
  D : sharedschedule/Interpolate Matrix(x)   matrix=com_piece.D  aMode=aMode
      settings: SourceProductName=Aerospace Blockset  SourceProductBaseCode=AE
  K : sharedschedule/Interpolate Matrix(x)   matrix=com_piece.K  aMode=aMode
      settings: SourceProductName=Aerospace Blockset  SourceProductBaseCode=AE
  Minus1 : Sum  Inputs=+-
  Prelookup : PreLookup  BreakpointsData=com_piece.Nl  BreakpointObject=Nl  ExtrapMethod=Linear  UseLastBreakpoint=on  DiagnosticForOutOfRangeInput=Warning
  S : sharedschedule/Interpolate Matrix(x)   matrix=com_piece.S  aMode=aMode
      settings: SourceProductName=Aerospace Blockset  SourceProductBaseCode=AE
  Selector : Selector  InputPortWidth=2  IndexOptions=Index vector (dialog)  Indices=[1]  OutputSizes=1
  kalman filter1 : Subsystem
  steadyOutput : sharedschedule/Interpolate Matrix(x)   matrix=com_piece.steadyOutput  aMode=aMode
      settings: SourceProductName=Aerospace Blockset  SourceProductBaseCode=AE
  steadyState : sharedschedule/Interpolate Matrix(x)   matrix=com_piece.steadyState  aMode=aMode
      settings: SourceProductName=Aerospace Blockset  SourceProductBaseCode=AE
  steadyinput : sharedschedule/Interpolate Matrix(x)   matrix=piece.steadyInput  aMode=aMode
      settings: SourceProductName=Aerospace Blockset  SourceProductBaseCode=AE
  Out1 : Outport
  Out2 : Outport  Port=2
  wires:
  Add/1 -> Out2/1
  steadyOutput/1 -> Add/2
  u/1 -> Minus1/1
  x0/1 -> kalman filter1/5(x0)
  A/1 -> kalman filter1/1(A)
  steadyinput/1 -> Minus1/2
  kalman filter1/1(X_es) -> Selector/1
  Minus1/1 -> kalman filter1/6(U)
  kalman filter1/2(Y_es) -> Out1/1, Add/1
  C/1 -> kalman filter1/3(C)
  steadyState/1 -> kalman filter1/7(Xtrim)
  Selector/1 -> Prelookup/1
  Prelookup/2 -> B/2, C/2, D/2, steadyOutput/2, steadyinput/2, K/2, S/2, steadyState/2, A/2
  B/1 -> kalman filter1/2(B)
  Prelookup/1 -> A/1, B/1, C/1, D/1, steadyOutput/1, steadyinput/1, steadyState/1, K/1, S/1
  D/1 -> kalman filter1/4(D)

== system kalman_estimate_MM/health_PWL ==
  In1 : Inport
  In3 : Inport  Port=2
  In4 : Inport  Port=3
  A : sharedschedule/Interpolate Matrix(x)   matrix=piece.A  aMode=aMode
      settings: SourceProductName=Aerospace Blockset  SourceProductBaseCode=AE
  Add : Sum
  B : sharedschedule/Interpolate Matrix(x)   matrix=piece.B  aMode=aMode
      settings: SourceProductName=Aerospace Blockset  SourceProductBaseCode=AE
  C : sharedschedule/Interpolate Matrix(x)   matrix=piece.C  aMode=aMode
      settings: SourceProductName=Aerospace Blockset  SourceProductBaseCode=AE
  D : sharedschedule/Interpolate Matrix(x)   matrix=piece.D  aMode=aMode
      settings: SourceProductName=Aerospace Blockset  SourceProductBaseCode=AE
  K_s : sharedschedule/Interpolate Matrix(x)   matrix=piece.K_s  aMode=aMode
      settings: SourceProductName=Aerospace Blockset  SourceProductBaseCode=AE
  L : sharedschedule/Interpolate Matrix(x)   matrix=piece.L  aMode=aMode
      settings: SourceProductName=Aerospace Blockset  SourceProductBaseCode=AE
  M : sharedschedule/Interpolate Matrix(x)   matrix=piece.M  aMode=aMode
      settings: SourceProductName=Aerospace Blockset  SourceProductBaseCode=AE
  MATLAB Function : MATLAB Function  TreatAsAtomicUnit=on
  Minus1 : Sum  Inputs=+-
  Prelookup : PreLookup  BreakpointsData=piece.Nl  BreakpointObject=Nl  ExtrapMethod=Linear  UseLastBreakpoint=on  DiagnosticForOutOfRangeInput=Warning
  S : sharedschedule/Interpolate Matrix(x)   matrix=piece.S_s  aMode=aMode
      settings: SourceProductName=Aerospace Blockset  SourceProductBaseCode=AE
  Selector : Selector  InputPortWidth=2  IndexOptions=Index vector (dialog)  Indices=[1]  OutputSizes=1
  kalman filter1 : Subsystem
  steadyOutput : sharedschedule/Interpolate Matrix(x)   matrix=piece.steadyOutput  aMode=aMode
      settings: SourceProductName=Aerospace Blockset  SourceProductBaseCode=AE
  steadyState : sharedschedule/Interpolate Matrix(x)   matrix=piece.steadyState  aMode=aMode
      settings: SourceProductName=Aerospace Blockset  SourceProductBaseCode=AE
  steadyinput : sharedschedule/Interpolate Matrix(x)   matrix=piece.steadyInput  aMode=aMode
      settings: SourceProductName=Aerospace Blockset  SourceProductBaseCode=AE
  Out1 : Outport
  Out2 : Outport  Port=2
  wires:
  D/1 -> kalman filter1/4(D)
  Prelookup/1 -> S/1, K_s/1, M/1, L/1, steadyState/1, steadyinput/1, steadyOutput/1, D/1, C/1, B/1, A/1
  In4/1 -> kalman filter1/11(P)
  B/1 -> kalman filter1/2(B)
  Prelookup/2 -> A/2, steadyState/2, S/2, K_s/2, M/2, L/2, steadyinput/2, steadyOutput/2, D/2, C/2, B/2
  Selector/1 -> Prelookup/1
  steadyState/1 -> kalman filter1/8(Xtrim)
  L/1 -> kalman filter1/9(L)
  C/1 -> kalman filter1/3(C)
  kalman filter1/2(Y_es) -> Add/1, Out1/1
  Minus1/1 -> kalman filter1/7(U)
  kalman filter1/1(X_es) -> Selector/1
  steadyinput/1 -> Minus1/2
  K_s/1 -> kalman filter1/5(K)
  A/1 -> kalman filter1/1(A)
  M/1 -> kalman filter1/10(M)
  In3/1 -> kalman filter1/6(x0)
  In1/1 -> Minus1/1
  steadyOutput/1 -> Add/2
  Add/1 -> Out2/1
  S/1 -> MATLAB Function/2(S)

== system kalman_estimate_MM/sen2_PIECE kalman2 ==
  u : Inport
  y : Inport  Port=2
  x0 : Inport  Port=3
  A : sharedschedule/Interpolate Matrix(x)   matrix=sen2_piece.A  aMode=aMode
      settings: SourceProductName=Aerospace Blockset  SourceProductBaseCode=AE
  B : sharedschedule/Interpolate Matrix(x)   matrix=sen2_piece.B  aMode=aMode
      settings: SourceProductName=Aerospace Blockset  SourceProductBaseCode=AE
  C : sharedschedule/Interpolate Matrix(x)   matrix=sen2_piece.C  aMode=aMode
      settings: SourceProductName=Aerospace Blockset  SourceProductBaseCode=AE
  D : sharedschedule/Interpolate Matrix(x)   matrix=sen2_piece.D  aMode=aMode
      settings: SourceProductName=Aerospace Blockset  SourceProductBaseCode=AE
  K_s : sharedschedule/Interpolate Matrix(x)   matrix=sen2_piece.K  aMode=aMode
      settings: SourceProductName=Aerospace Blockset  SourceProductBaseCode=AE
  MATLAB Function : MATLAB Function  TreatAsAtomicUnit=on
  Minus1 : Sum  Inputs=+-
  Minus5 : Sum  Inputs=+-
  Prelookup : PreLookup  BreakpointsData=sen2_piece.Nl  BreakpointObject=Nl  ExtrapMethod=Linear  UseLastBreakpoint=on  DiagnosticForOutOfRangeInput=Warning
  S : sharedschedule/Interpolate Matrix(x)   matrix=sen2_piece.S  aMode=aMode
      settings: SourceProductName=Aerospace Blockset  SourceProductBaseCode=AE
  Selector : Selector  InputPortWidth=2  IndexOptions=Index vector (dialog)  Indices=[1]  OutputSizes=1
  kalman filter1 : Subsystem
  steadyOutput : sharedschedule/Interpolate Matrix(x)   matrix=sen2_piece.steadyOutput  aMode=aMode
      settings: SourceProductName=Aerospace Blockset  SourceProductBaseCode=AE
  steadyState : sharedschedule/Interpolate Matrix(x)   matrix=sen2_piece.steadyState  aMode=aMode
      settings: SourceProductName=Aerospace Blockset  SourceProductBaseCode=AE
  steadyinput : sharedschedule/Interpolate Matrix(x)   matrix=sen2_piece.steadyInput  aMode=aMode
      settings: SourceProductName=Aerospace Blockset  SourceProductBaseCode=AE
  Out1 : Outport
  Out2 : Outport  Port=2
  Out3 : Outport  Port=3
  wires:
  kalman filter1/3(Y_error) -> MATLAB Function/1(err), Out2/1
  u/1 -> Minus1/1
  y/1 -> Minus5/1
  x0/1 -> kalman filter1/6(x0)
  A/1 -> kalman filter1/1(A)
  steadyOutput/1 -> Minus5/2
  K_s/1 -> kalman filter1/5(K)
  steadyinput/1 -> Minus1/2
  kalman filter1/1(X_es) -> Selector/1
  Minus1/1 -> kalman filter1/8(U)
  kalman filter1/2(Y_es) -> Out1/1
  Minus5/1 -> kalman filter1/7(Y)
  C/1 -> kalman filter1/3(C)
  steadyState/1 -> kalman filter1/9(Xtrim)
  Selector/1 -> Prelookup/1
  Prelookup/2 -> B/2, C/2, D/2, steadyOutput/2, steadyinput/2, K_s/2, S/2, steadyState/2, A/2
  B/1 -> kalman filter1/2(B)
  Prelookup/1 -> A/1, B/1, C/1, D/1, steadyOutput/1, steadyinput/1, steadyState/1, K_s/1, S/1
  D/1 -> kalman filter1/4(D)
  S/1 -> MATLAB Function/2(S)
  MATLAB Function/1(y) -> Out3/1

== system kalman_estimate_MM/sen2_PWL ==
  u : Inport
  x0 : Inport  Port=2
  A : sharedschedule/Interpolate Matrix(x)   matrix=sen2_piece.A  aMode=aMode
      settings: SourceProductName=Aerospace Blockset  SourceProductBaseCode=AE
  Add : Sum
  B : sharedschedule/Interpolate Matrix(x)   matrix=sen2_piece.B  aMode=aMode
      settings: SourceProductName=Aerospace Blockset  SourceProductBaseCode=AE
  C : sharedschedule/Interpolate Matrix(x)   matrix=sen2_piece.C  aMode=aMode
      settings: SourceProductName=Aerospace Blockset  SourceProductBaseCode=AE
  D : sharedschedule/Interpolate Matrix(x)   matrix=sen2_piece.D  aMode=aMode
      settings: SourceProductName=Aerospace Blockset  SourceProductBaseCode=AE
  K : sharedschedule/Interpolate Matrix(x)   matrix=sen2_piece.K  aMode=aMode
      settings: SourceProductName=Aerospace Blockset  SourceProductBaseCode=AE
  Minus1 : Sum  Inputs=+-
  Prelookup : PreLookup  BreakpointsData=sen2_piece.Nl  BreakpointObject=Nl  ExtrapMethod=Linear  UseLastBreakpoint=on  DiagnosticForOutOfRangeInput=Warning
  S : sharedschedule/Interpolate Matrix(x)   matrix=sen2_piece.S  aMode=aMode
      settings: SourceProductName=Aerospace Blockset  SourceProductBaseCode=AE
  Selector : Selector  InputPortWidth=2  IndexOptions=Index vector (dialog)  Indices=[1]  OutputSizes=1
  kalman filter1 : Subsystem
  steadyOutput : sharedschedule/Interpolate Matrix(x)   matrix=sen2_piece.steadyOutput  aMode=aMode
      settings: SourceProductName=Aerospace Blockset  SourceProductBaseCode=AE
  steadyState : sharedschedule/Interpolate Matrix(x)   matrix=sen2_piece.steadyState  aMode=aMode
      settings: SourceProductName=Aerospace Blockset  SourceProductBaseCode=AE
  steadyinput : sharedschedule/Interpolate Matrix(x)   matrix=sen2_piece.steadyInput  aMode=aMode
      settings: SourceProductName=Aerospace Blockset  SourceProductBaseCode=AE
  Out1 : Outport
  Out2 : Outport  Port=2
  wires:
  Add/1 -> Out2/1
  steadyOutput/1 -> Add/2
  u/1 -> Minus1/1
  x0/1 -> kalman filter1/5(x0)
  A/1 -> kalman filter1/1(A)
  steadyinput/1 -> Minus1/2
  kalman filter1/1(X_es) -> Selector/1
  Minus1/1 -> kalman filter1/6(U)
  kalman filter1/2(Y_es) -> Out1/1, Add/1
  C/1 -> kalman filter1/3(C)
  steadyState/1 -> kalman filter1/7(Xtrim)
  Selector/1 -> Prelookup/1
  Prelookup/2 -> B/2, D/2, steadyOutput/2, steadyinput/2, K/2, S/2, steadyState/2, C/2, A/2
  B/1 -> kalman filter1/2(B)
  Prelookup/1 -> A/1, B/1, D/1, steadyOutput/1, steadyinput/1, steadyState/1, K/1, S/1, C/1
  D/1 -> kalman filter1/4(D)

== system kalman_estimate_MM/sen3_PIECE kalman1 ==
  u : Inport
  y : Inport  Port=2
  x0 : Inport  Port=3
  A : sharedschedule/Interpolate Matrix(x)   matrix=sen3_piece.A  aMode=aMode
      settings: SourceProductName=Aerospace Blockset  SourceProductBaseCode=AE
  B : sharedschedule/Interpolate Matrix(x)   matrix=sen3_piece.B  aMode=aMode
      settings: SourceProductName=Aerospace Blockset  SourceProductBaseCode=AE
  C : sharedschedule/Interpolate Matrix(x)   matrix=sen3_piece.C  aMode=aMode
      settings: SourceProductName=Aerospace Blockset  SourceProductBaseCode=AE
  Constant : Constant  Value=[0,0,0.03,0,0,0,0,0,0,0]'  VectorParams1D=off
  D : sharedschedule/Interpolate Matrix(x)   matrix=sen3_piece.D  aMode=aMode
      settings: SourceProductName=Aerospace Blockset  SourceProductBaseCode=AE
  K_s : sharedschedule/Interpolate Matrix(x)   matrix=sen3_piece.K  aMode=aMode
      settings: SourceProductName=Aerospace Blockset  SourceProductBaseCode=AE
  MATLAB Function : MATLAB Function  TreatAsAtomicUnit=on
  Minus1 : Sum  Inputs=+-
  Minus2 : Sum
  Minus5 : Sum  Inputs=+-
  Prelookup : PreLookup  BreakpointsData=sen3_piece.Nl  BreakpointObject=Nl  ExtrapMethod=Linear  UseLastBreakpoint=on  DiagnosticForOutOfRangeInput=Warning
  S : sharedschedule/Interpolate Matrix(x)   matrix=sen3_piece.S  aMode=aMode
      settings: SourceProductName=Aerospace Blockset  SourceProductBaseCode=AE
  Selector : Selector  InputPortWidth=2  IndexOptions=Index vector (dialog)  Indices=[1]  OutputSizes=1
  kalman filter1 : Subsystem
  steadyOutput : sharedschedule/Interpolate Matrix(x)   matrix=sen3_piece.steadyOutput  aMode=aMode
      settings: SourceProductName=Aerospace Blockset  SourceProductBaseCode=AE
  steadyState : sharedschedule/Interpolate Matrix(x)   matrix=sen3_piece.steadyState  aMode=aMode
      settings: SourceProductName=Aerospace Blockset  SourceProductBaseCode=AE
  steadyinput : sharedschedule/Interpolate Matrix(x)   matrix=sen3_piece.steadyInput  aMode=aMode
      settings: SourceProductName=Aerospace Blockset  SourceProductBaseCode=AE
  Out1 : Outport
  Out2 : Outport  Port=2
  Out3 : Outport  Port=3
  wires:
  MATLAB Function/1(y) -> Out3/1
  S/1 -> MATLAB Function/2(S)
  D/1 -> kalman filter1/4(D)
  Prelookup/1 -> S/1, K_s/1, steadyState/1, steadyinput/1, steadyOutput/1, D/1, C/1, B/1, A/1
  B/1 -> kalman filter1/2(B)
  Prelookup/2 -> A/2, steadyState/2, S/2, K_s/2, steadyinput/2, steadyOutput/2, D/2, C/2, B/2
  Selector/1 -> Prelookup/1
  steadyState/1 -> kalman filter1/9(Xtrim)
  C/1 -> kalman filter1/3(C)
  Minus5/1 -> kalman filter1/7(Y)
  kalman filter1/2(Y_es) -> Out1/1
  Minus1/1 -> kalman filter1/8(U)
  kalman filter1/1(X_es) -> Selector/1
  steadyinput/1 -> Minus1/2
  K_s/1 -> kalman filter1/5(K)
  A/1 -> kalman filter1/1(A)
  x0/1 -> kalman filter1/6(x0)
  y/1 -> Minus5/1
  u/1 -> Minus1/1
  kalman filter1/3(Y_error) -> Out2/1, MATLAB Function/1(err)
  steadyOutput/1 -> Minus2/1
  Minus2/1 -> Minus5/2
  Constant/1 -> Minus2/2

== system kalman_estimate_MM/sen3_PIECE kalman3 ==
  u : Inport
  y : Inport  Port=2
  x0 : Inport  Port=3
  A : sharedschedule/Interpolate Matrix(x)   matrix=sen3_piece.A  aMode=aMode
      settings: SourceProductName=Aerospace Blockset  SourceProductBaseCode=AE
  B : sharedschedule/Interpolate Matrix(x)   matrix=sen3_piece.B  aMode=aMode
      settings: SourceProductName=Aerospace Blockset  SourceProductBaseCode=AE
  C : sharedschedule/Interpolate Matrix(x)   matrix=sen3_piece.C  aMode=aMode
      settings: SourceProductName=Aerospace Blockset  SourceProductBaseCode=AE
  D : sharedschedule/Interpolate Matrix(x)   matrix=sen3_piece.D  aMode=aMode
      settings: SourceProductName=Aerospace Blockset  SourceProductBaseCode=AE
  K_s : sharedschedule/Interpolate Matrix(x)   matrix=sen3_piece.K  aMode=aMode
      settings: SourceProductName=Aerospace Blockset  SourceProductBaseCode=AE
  MATLAB Function : MATLAB Function  TreatAsAtomicUnit=on
  Minus1 : Sum  Inputs=+-
  Minus5 : Sum  Inputs=+-
  Prelookup : PreLookup  BreakpointsData=sen3_piece.Nl  BreakpointObject=Nl  ExtrapMethod=Linear  UseLastBreakpoint=on  DiagnosticForOutOfRangeInput=Warning
  S : sharedschedule/Interpolate Matrix(x)   matrix=sen3_piece.S  aMode=aMode
      settings: SourceProductName=Aerospace Blockset  SourceProductBaseCode=AE
  Selector : Selector  InputPortWidth=2  IndexOptions=Index vector (dialog)  Indices=[1]  OutputSizes=1
  kalman filter1 : Subsystem
  steadyOutput : sharedschedule/Interpolate Matrix(x)   matrix=sen3_piece.steadyOutput  aMode=aMode
      settings: SourceProductName=Aerospace Blockset  SourceProductBaseCode=AE
  steadyState : sharedschedule/Interpolate Matrix(x)   matrix=sen3_piece.steadyState  aMode=aMode
      settings: SourceProductName=Aerospace Blockset  SourceProductBaseCode=AE
  steadyinput : sharedschedule/Interpolate Matrix(x)   matrix=sen3_piece.steadyInput  aMode=aMode
      settings: SourceProductName=Aerospace Blockset  SourceProductBaseCode=AE
  Out1 : Outport
  Out2 : Outport  Port=2
  Out3 : Outport  Port=3
  wires:
  kalman filter1/3(Y_error) -> MATLAB Function/1(err), Out2/1
  u/1 -> Minus1/1
  y/1 -> Minus5/1
  x0/1 -> kalman filter1/6(x0)
  A/1 -> kalman filter1/1(A)
  steadyOutput/1 -> Minus5/2
  K_s/1 -> kalman filter1/5(K)
  steadyinput/1 -> Minus1/2
  kalman filter1/1(X_es) -> Selector/1
  Minus1/1 -> kalman filter1/8(U)
  kalman filter1/2(Y_es) -> Out1/1
  Minus5/1 -> kalman filter1/7(Y)
  C/1 -> kalman filter1/3(C)
  steadyState/1 -> kalman filter1/9(Xtrim)
  Selector/1 -> Prelookup/1
  Prelookup/2 -> B/2, C/2, D/2, steadyOutput/2, steadyinput/2, K_s/2, S/2, steadyState/2, A/2
  B/1 -> kalman filter1/2(B)
  Prelookup/1 -> A/1, B/1, C/1, D/1, steadyOutput/1, steadyinput/1, steadyState/1, K_s/1, S/1
  D/1 -> kalman filter1/4(D)
  S/1 -> MATLAB Function/2(S)
  MATLAB Function/1(y) -> Out3/1

== system kalman_estimate_MM/sen3_PWL ==
  u : Inport
  x0 : Inport  Port=2
  A : sharedschedule/Interpolate Matrix(x)   matrix=sen3_piece.A  aMode=aMode
      settings: SourceProductName=Aerospace Blockset  SourceProductBaseCode=AE
  Add : Sum
  B : sharedschedule/Interpolate Matrix(x)   matrix=sen3_piece.B  aMode=aMode
      settings: SourceProductName=Aerospace Blockset  SourceProductBaseCode=AE
  C : sharedschedule/Interpolate Matrix(x)   matrix=sen3_piece.C  aMode=aMode
      settings: SourceProductName=Aerospace Blockset  SourceProductBaseCode=AE
  D : sharedschedule/Interpolate Matrix(x)   matrix=sen3_piece.D  aMode=aMode
      settings: SourceProductName=Aerospace Blockset  SourceProductBaseCode=AE
  K : sharedschedule/Interpolate Matrix(x)   matrix=sen3_piece.K  aMode=aMode
      settings: SourceProductName=Aerospace Blockset  SourceProductBaseCode=AE
  Minus1 : Sum  Inputs=+-
  Prelookup : PreLookup  BreakpointsData=sen3_piece.Nl  BreakpointObject=Nl  ExtrapMethod=Linear  UseLastBreakpoint=on  DiagnosticForOutOfRangeInput=Warning
  S : sharedschedule/Interpolate Matrix(x)   matrix=sen3_piece.S  aMode=aMode
      settings: SourceProductName=Aerospace Blockset  SourceProductBaseCode=AE
  Selector : Selector  InputPortWidth=2  IndexOptions=Index vector (dialog)  Indices=[1]  OutputSizes=1
  kalman filter1 : Subsystem
  steadyOutput : sharedschedule/Interpolate Matrix(x)   matrix=sen3_piece.steadyOutput  aMode=aMode
      settings: SourceProductName=Aerospace Blockset  SourceProductBaseCode=AE
  steadyState : sharedschedule/Interpolate Matrix(x)   matrix=sen3_piece.steadyState  aMode=aMode
      settings: SourceProductName=Aerospace Blockset  SourceProductBaseCode=AE
  steadyinput : sharedschedule/Interpolate Matrix(x)   matrix=sen3_piece.steadyInput  aMode=aMode
      settings: SourceProductName=Aerospace Blockset  SourceProductBaseCode=AE
  Out1 : Outport
  Out2 : Outport  Port=2
  wires:
  Add/1 -> Out2/1
  steadyOutput/1 -> Add/2
  u/1 -> Minus1/1
  x0/1 -> kalman filter1/5(x0)
  A/1 -> kalman filter1/1(A)
  steadyinput/1 -> Minus1/2
  kalman filter1/1(X_es) -> Selector/1
  Minus1/1 -> kalman filter1/6(U)
  kalman filter1/2(Y_es) -> Out1/1, Add/1
  C/1 -> kalman filter1/3(C)
  steadyState/1 -> kalman filter1/7(Xtrim)
  Selector/1 -> Prelookup/1
  Prelookup/2 -> B/2, D/2, steadyOutput/2, steadyinput/2, K/2, S/2, steadyState/2, C/2, A/2
  B/1 -> kalman filter1/2(B)
  Prelookup/1 -> A/1, B/1, D/1, steadyOutput/1, steadyinput/1, steadyState/1, K/1, S/1, C/1
  D/1 -> kalman filter1/4(D)
